simulink model "L1_C_FULL"  (R2020a)
settings: Solver=VariableStepAuto  StartTime=0.0  StopTime=10.0  RelTol=1e-3
settings Model: Creator=fbi  LastModifiedBy=fbi

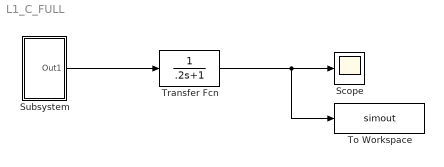
== system L1_C_FULL ==
  Scope : Scope
  Subsystem : Subsystem
  To Workspace : ToWorkspace  VariableName=simout  SaveFormat=Timeseries  SampleTime=-1
  Transfer Fcn : TransferFcn  Denominator=[.2 1]
  wires:
  Subsystem/1(Out1) -> Transfer Fcn/1
  Transfer Fcn/1 -> To Workspace/1, Scope/1

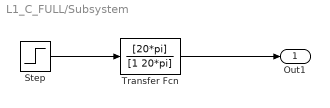
== system L1_C_FULL/Subsystem ==
  Step : Step  Time=0  SampleTime=0
  Transfer Fcn : TransferFcn  Numerator=[20*pi]  Denominator=[1 20*pi]
  Out1 : Outport
  wires:
  Step/1 -> Transfer Fcn/1
  Transfer Fcn/1 -> Out1/1
